simulink model "KALMAN"  (R2019b)
settings: Solver=VariableStepAuto  StartTime=0.0  StopTime=10.0  RelTol=1e-3
values from neighbouring files (symbols this model uses):
  A = [0      1              0           0 ... (first row only)    [LQG.m]    (also in State_Space.m; inverted_pendulum.m; rscale.m = a)
  B = [     0 ... (first row only)    [LQG.m]    (also in State_Space.m; inverted_pendulum.m; rscale.m = b)
  C = [1 0 0 0 ... (first row only)    [LQG.m]    (also in PID.m = pid(Kp,Ki,Kd); State_Space.m; frequency_domain.m = K*(((s+1)*(s+0.7491))/s); inverted_pendulum.m)
  D = [0 ... (first row only)    [LQG.m]    (also in State_Space.m; inverted_pendulum.m; rscale.m = d)
  K = lqr(A,B,Q,R)    [LQG.m]    (also in State_Space.m; frequency_domain.m = 35; root_locus_method.m = 20; rscale.m = k)
  Nbar = rscale(sys_ss,K)    [State_Space.m]    (also in rscale.m = Nu + K*Nx)
undefined symbols (not defined in the file or in its folder): Ke
settings Model: Creator=Khojasteh Mirza  LastModifiedBy=Khojasteh Mirza

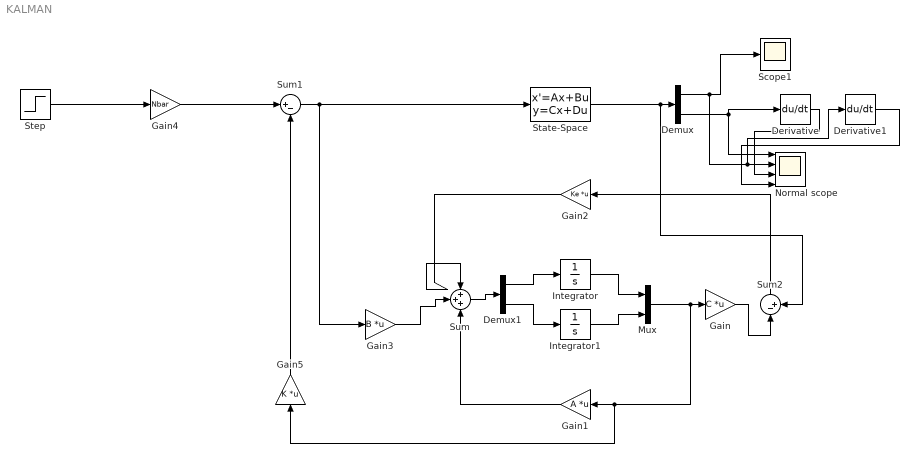
== system KALMAN ==
  Demux : Demux  Outputs=2
  Demux1 : Demux  Outputs=2
  Derivative : Derivative
  Derivative1 : Derivative
  Gain : Gain  Gain=C  Multiplication=Matrix(K*u)
  Gain1 : Gain  Gain=A  Multiplication=Matrix(K*u)
  Gain2 : Gain  Gain=Ke  Multiplication=Matrix(K*u)
  Gain3 : Gain  Gain=B  Multiplication=Matrix(K*u)
  Gain4 : Gain  Gain=Nbar
  Gain5 : Gain  Gain=K  Multiplication=Matrix(K*u)
  Integrator : Integrator
  Integrator1 : Integrator
  Mux : Mux  Inputs=2
  "Normal scope " : Scope  NumInputPorts=4
  Scope1 : Scope
  State-Space : StateSpace  A=A  B=B  C=C  D=D  InitialCondition=0
  Step : Step  After=0.5  SampleTime=0
  Sum : Sum  Inputs=3
  Sum1 : Sum  Inputs=|+-
  Sum2 : Sum  Inputs=|-+
  wires:
  State-Space/1 -> Sum2/2, Demux/1
  Demux/2 -> "Normal scope "/1, Derivative/1
  Demux/1 -> Derivative1/1, "Normal scope "/2, Scope1/1
  Sum1/1 -> Gain3/1, State-Space/1
  Sum/1 -> Demux1/1
  Demux1/1 -> Integrator/1
  Demux1/2 -> Integrator1/1
  Integrator/1 -> Mux/1
  Integrator1/1 -> Mux/2
  Mux/1 -> Gain5/1, Gain1/1, Gain/1
  Gain/1 -> Sum2/1
  Sum2/1 -> Gain2/1
  Gain2/1 -> Sum/1
  Gain3/1 -> Sum/2
  Gain1/1 -> Sum/3
  Step/1 -> Gain4/1
  Gain5/1 -> Sum1/2
  Gain4/1 -> Sum1/1
  Derivative/1 -> "Normal scope "/3
  Derivative1/1 -> "Normal scope "/4
